simulink model "Tank_reglering"  (R2017b)
settings: Solver=VariableStepAuto  StartTime=0.0  StopTime=inf  RelTol=1e-3
values from neighbouring files (symbols this model uses):
  H = [2.5 5.4 6.9 8.2 9.6 13.1 15.5]    [tank.m]
  Y = [0.10 2.33 3.43 4.49 5.54 8.22 9.91]    [tank.m]
libraries: Tank_bib x1
settings Model: Creator=Oliver  LastModifiedBy=Oliver

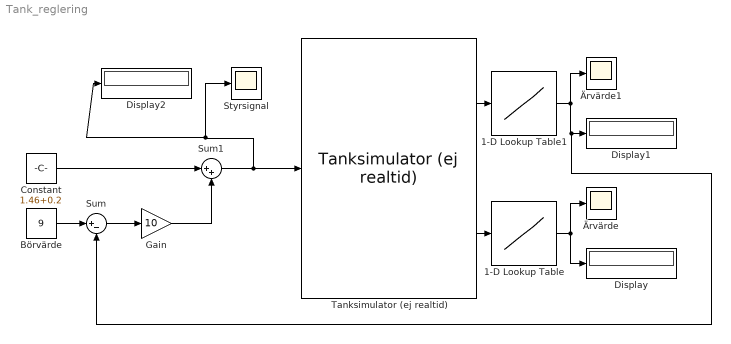
== system Tank_reglering ==
  1-D Lookup Table : Lookup_n-D  NumberOfTableDimensions=1  BreakpointsForDimension1=Y  Table=H  InternalRulePriority=Speed  RndMeth=Simplest  InputSameDT=on
  1-D Lookup Table1 : Lookup_n-D  NumberOfTableDimensions=1  BreakpointsForDimension1=Y  Table=H  InternalRulePriority=Speed  RndMeth=Simplest  InputSameDT=on
  Börvärde : Constant  Value=9
  Constant : Constant  Value=1.46+0.2
  Display : Display
      settings: Format=bank
  Display1 : Display
      settings: Format=bank
  Display2 : Display
  Gain : Gain  Gain=10
  Styrsignal : Scope
  Sum : Sum  Inputs=|+-
  Sum1 : Sum  Inputs=|++
  Tanksimulator (ej realtid) : Tank_bib/Tanksimulator (ej realtid)  valve_opening=0  plug=off
  Ärvärde : Scope
  Ärvärde1 : Scope
  wires:
  1-D Lookup Table/1 -> Ärvärde/1, Display/1
  Tanksimulator (ej realtid)/2 -> 1-D Lookup Table/1
  1-D Lookup Table1/1 -> Display1/1, Sum/2, Ärvärde1/1
  Tanksimulator (ej realtid)/1 -> 1-D Lookup Table1/1
  Börvärde/1 -> Sum/1
  Sum/1 -> Gain/1
  Gain/1 -> Sum1/2
  Sum1/1 -> Tanksimulator (ej realtid)/1, Display2/1, Styrsignal/1
  Constant/1 -> Sum1/1
